simulink library "plan_lib"  (R2018b)
settings: Solver=VariableStepAuto  StartTime=0.0  StopTime=10.0  RelTol=1e-3
settings Model: Creator=Ybeyer  LastModifiedBy=yannic
settings DebuggingCC: LibraryContextMissingDiagnostic=none
settings SFSimCC: SimUseLocalCustomCode=off
settings RTWCC: RTWUseLocalCustomCode=off
settings CodeAppCC: StateflowObjectComments=on

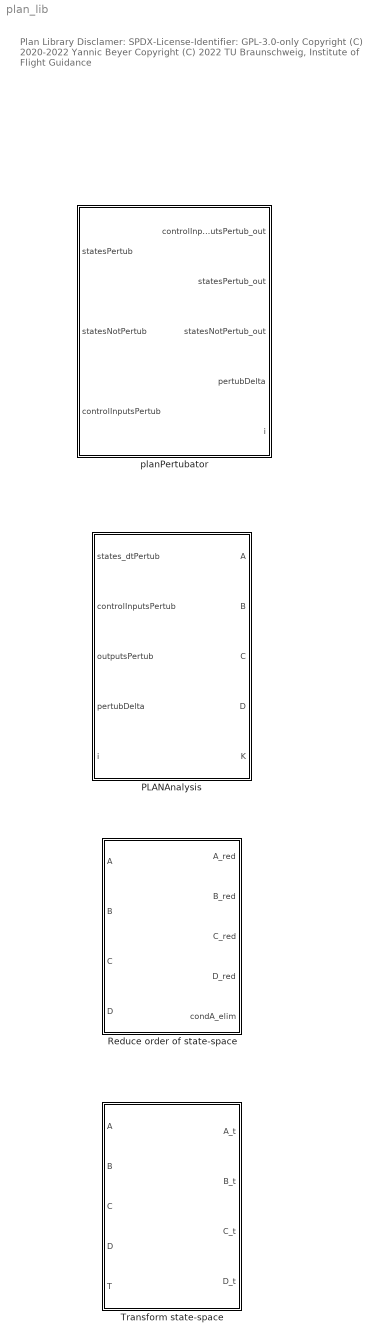
== system plan_lib ==
  note: Plan Library
      |
      | Disclamer:
      | SPDX-License-Identifier: GPL-3.0-only
      |
      | Copyright (C) 2020-2022 Yannic Beyer
      | Copyright (C) 2022 TU Braunschweig, Institute of Flight Guidance
  PLANAnalysis : MATLAB Function  TreatAsAtomicUnit=on  SystemSampleTime=1/400
  Reduce order of state-space : MATLAB Function  TreatAsAtomicUnit=on
  Transform state-space : MATLAB Function  TreatAsAtomicUnit=on
  planPertubator : Subsystem  mask{plantStateDelta=0, controlInputsDelta=0}
      mask prompts: plantStateDelta "State pertubation delta (struct)"; controlInputsDelta "Control input pertubation delta (struct)"

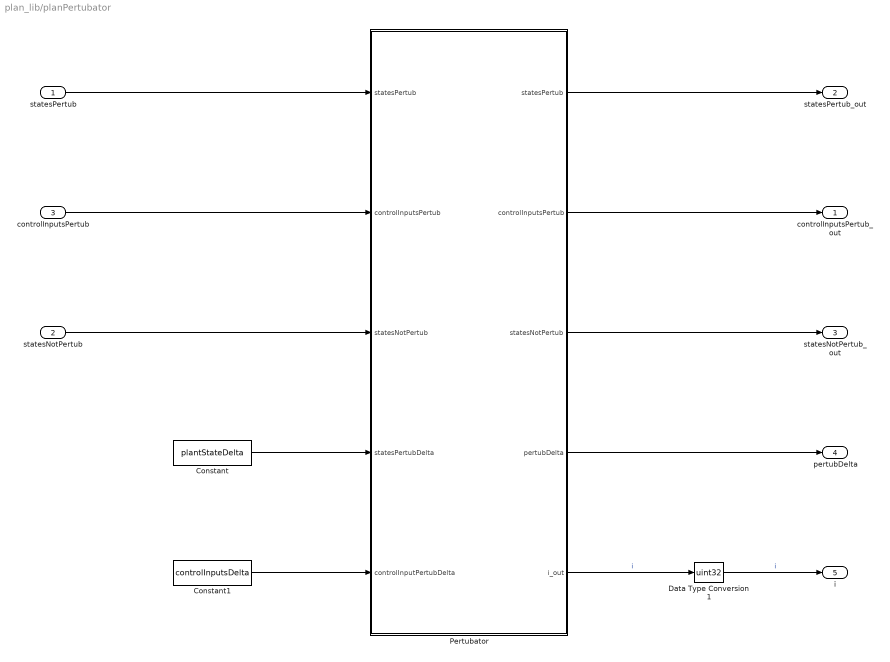
== system plan_lib/planPertubator ==
  statesPertub : Inport
  statesNotPertub : Inport  Port=2
  controlInputsPertub : Inport  Port=3
  Constant : Constant  Value=plantStateDelta  OutDataTypeStr=Bus: integratorBus  SampleTime=-1
  Constant1 : Constant  Value=controlInputsDelta  OutDataTypeStr=Bus: controlInputsBus  SampleTime=-1
  Data Type Conversion1 : DataTypeConversion  OutDataTypeStr=uint32
  Pertubator : MATLAB Function  TreatAsAtomicUnit=on  SystemSampleTime=1/400
  controlInputsPertub_out : Outport
  statesPertub_out : Outport  Port=2
  statesNotPertub_out : Outport  Port=3
  pertubDelta : Outport  Port=4
  i : Outport  Port=5
  wires:
  statesPertub/1 -> Pertubator/1("statesPertub ")
  Pertubator/5(i_out) -> Data Type Conversion1/1  "i"
  Pertubator/1(statesPertub) -> statesPertub_out/1
  Pertubator/3(statesNotPertub) -> statesNotPertub_out/1
  controlInputsPertub/1 -> Pertubator/2("controlInputsPertub ")
  Constant/1 -> Pertubator/4(statesPertubDelta)
  Constant1/1 -> Pertubator/5(controlInputPertubDelta)
  Data Type Conversion1/1 -> i/1  "i"
  Pertubator/2(controlInputsPertub) -> controlInputsPertub_out/1
  statesNotPertub/1 -> Pertubator/3("statesNotPertub ")
  Pertubator/4(pertubDelta) -> pertubDelta/1

== matlab function plan_lib/Reduce order of state-space ==
  data: A input; A_red output; B input; C input; D input; B_red output; C_red output; D_red output; condA_elim output; elim parameter boolean
function [ A_red, B_red, C_red, D_red, condA_elim ] = fcn( ...
    A, B, C, D, elim ) %#codegen
[ A_red, B_red, C_red, D_red, condA_elim ] = modredEmb2( ...
    A, B, C, D, elim );
end

== matlab function plan_lib/PLANAnalysis ==
  data: states_dtPertub input; A output; controlInputsPertub input; B output; C output; D output; K output; outputsPertub input; pertubDelta input; i input
function [ A, B, C, D, K ] = fcn( states_dtPertub, controlInputsPertub, ...
    outputsPertub, pertubDelta, i ) %#codegen
[ A, B, C, D, K ] = planAnalysis( states_dtPertub, controlInputsPertub, ...
    outputsPertub, pertubDelta, i );
end

== matlab function plan_lib/Transform state-space ==
  data: A input; A_t output; B input; C input; D input; T input; B_t output; C_t output; D_t output
function [ A_t, B_t, C_t, D_t ] = fcn( A, B, C, D, T ) %#codegen
[ A_t, B_t, C_t, D_t ] = transformStateSpace( A, B, C, D, T );
end

== matlab function plan_lib/planPertubator/Pertubator ==
  data: statesPertub output; controlInputsPertub output; statesNotPertub output; pertubDelta output; statesPertub input Bus: integratorBus; controlInputsPertub input Bus: controlInputsBus; i_out output size=1; statesNotPertub input Bus: integratorBus; statesPertubDelta input Bus: integratorBus; controlInputPertubDelta input Bus: controlInputsBus
function [ statesPertub, controlInputsPertub, statesNotPertub, ...
    pertubDelta, i_out ]...
    = pertubator( statesPertub, controlInputsPertub, statesNotPertub, ...
    statesPertubDelta, controlInputPertubDelta ) %#codegen
[ statesPertub, controlInputsPertub, statesNotPertub, ...
    pertubDelta, i_out ]...
    = planPertubator( statesPertub, controlInputsPertub, statesNotPertub, ...
    statesPertubDelta, controlInputPertubDelta );
end
